simulink library "Simple_lib"  (R2018b)
settings: Solver=ode45  StartTime=0.0  StopTime=10.0  RelTol=1e-3  EnableMultiTasking=on
undefined symbols (not defined in the file or in its folder): Acceptance, beta, C, C_J, C_P, c_wall, dGain, DiscIntNeverNeededParam, Duplex, Electrical_lib, grab, h_fe, i, i3, K_T, Kman, KmanCE, mu_s, n_rev, R_arm, Simplex, systemTs, tau_0, TinIC, Ts, w_0, wallMass, Watch_lib
libraries: $bdroot x407, PlantUtilityBlockset_lib x30, peGeneralControl x22, simulink x11
(part 11 of 14)

== system Simple_lib/Electrical/B2/C ==
  1/C_J : Gain  Gain=1/C_J
  Discrete-Time Integrator1 : DiscreteIntegrator  gainval=1  SampleTime=Ts  ICPrevOutput=DiscIntNeverNeededParam  ICPrevScaledInput=DiscIntNeverNeededParam
  Duplex : Subsystem  AncestorBlock=Electrical_lib/Duplex  InitFcn=bond
      mask Display:
      | plot([1 1], [2 -2])
      | plot([0 1],[0 1])
  J1 : Outport
  wires:
  Discrete-Time Integrator1/1 -> Duplex/1(potential)
  1/C_J/1 -> Discrete-Time Integrator1/1
  Duplex/2(flow) -> 1/C_J/1
  Duplex/1(duplex) -> J1/1

== system Simple_lib/Electrical/B2/E ==
  In1 : Inport
  Constant : Constant  Value=1.5
  Duplex : Subsystem  AncestorBlock=Electrical_lib/Duplex  InitFcn=bond
      mask Display:
      | plot([1 1], [2 -2])
      | plot([0 1],[0 1])
  Simplex : Subsystem  AncestorBlock=Electrical_lib/Simplex  InitFcn=bond
      mask Display:
      | color('white')
      | plot([0 1], [2 2])
      | plot([0 1], [-2 -2])
      | color('black')
      | %patch([0 1 0 0], [0 1 2 0], [0 0 0])
      | plot([0 0], [2 -2])
      | %patch([0 1 1 0 0], [0 0 -2 -2 0], [0 0 0])
      | %patch([-1 0 0 -1 -1], [-2 -2 2 2 -2], [0 0 0])
      | plot([0 1],[1 0])
  Sum : Sum  Inputs=|++
  Out1 : Outport
  wires:
  In1/1 -> Simplex/1(duplex)
  Sum/1 -> Duplex/1(potential)
  Constant/1 -> Sum/2
  Duplex/2(flow) -> Simplex/2(In2)
  Simplex/1(simplex) -> Sum/1
  Duplex/1(duplex) -> Out1/1

== system Simple_lib/Electrical/B2/L ==
  In1 : Inport
  In2 : Inport  Port=2
  1/L : Gain  Gain=-1/1e-1
  1/R2 : Gain  Gain=-1
  1/R3 : Gain  Gain=-1
  Discrete-Time Integrator1 : DiscreteIntegrator  gainval=1  SampleTime=Ts  ICPrevOutput=DiscIntNeverNeededParam  ICPrevScaledInput=DiscIntNeverNeededParam
  Simplex : Subsystem  AncestorBlock=Electrical_lib/Simplex  InitFcn=bond
      mask Display:
      | color('white')
      | plot([0 1], [2 2])
      | plot([0 1], [-2 -2])
      | color('black')
      | %patch([0 1 0 0], [0 1 2 0], [0 0 0])
      | plot([0 0], [2 -2])
      | %patch([0 1 1 0 0], [0 0 -2 -2 0], [0 0 0])
      | %patch([-1 0 0 -1 -1], [-2 -2 2 2 -2], [0 0 0])
      | plot([0 1],[1 0])
  Simplex1 : Subsystem  AncestorBlock=Electrical_lib/Simplex  InitFcn=bond
      mask Display:
      | color('white')
      | plot([0 1], [2 2])
      | plot([0 1], [-2 -2])
      | color('black')
      | %patch([0 1 0 0], [0 1 2 0], [0 0 0])
      | plot([0 0], [2 -2])
      | %patch([0 1 1 0 0], [0 0 -2 -2 0], [0 0 0])
      | %patch([-1 0 0 -1 -1], [-2 -2 2 2 -2], [0 0 0])
      | plot([0 1],[1 0])
  Sum : Sum  Inputs=+|+
  wires:
  In1/1 -> Simplex/1(duplex)
  In2/1 -> Simplex1/1(duplex)
  Sum/1 -> Discrete-Time Integrator1/1
  1/R2/1 -> Sum/1
  1/L/1 -> 1/R3/1, Simplex/2(In2)
  Discrete-Time Integrator1/1 -> 1/L/1
  1/R3/1 -> Simplex1/2(In2)
  Simplex1/1(simplex) -> Sum/2
  Simplex/1(simplex) -> 1/R2/1

== system Simple_lib/Electrical/B2/R0 ==
  In1 : Inport
  Duplex : Subsystem  AncestorBlock=Electrical_lib/Duplex  InitFcn=bond
      mask Display:
      | plot([1 1], [2 -2])
      | plot([0 1],[0 1])
  Gain : Gain  Gain=-1
  Simplex : Subsystem  AncestorBlock=Electrical_lib/Simplex  InitFcn=bond
      mask Display:
      | color('white')
      | plot([0 1], [2 2])
      | plot([0 1], [-2 -2])
      | color('black')
      | %patch([0 1 0 0], [0 1 2 0], [0 0 0])
      | plot([0 0], [2 -2])
      | %patch([0 1 1 0 0], [0 0 -2 -2 0], [0 0 0])
      | %patch([-1 0 0 -1 -1], [-2 -2 2 2 -2], [0 0 0])
      | plot([0 1],[1 0])
  Sum : Sum  Inputs=|++
  resistance : Gain  Gain=R
  Out1 : Outport
  wires:
  Sum/1 -> Duplex/1(potential)
  Gain/1 -> Sum/2
  resistance/1 -> Gain/1
  Duplex/1(duplex) -> Out1/1
  In1/1 -> Simplex/1(duplex)
  Simplex/1(simplex) -> Sum/1
  Duplex/2(flow) -> Simplex/2(In2), resistance/1

== system Simple_lib/Electrical/BiGain/_out ==
  note: {\bf\_out - buses out and logs the signals from the generic {\itOutflow} block}
      |
      | The init function {\itinit\_out} sets up the logging.
  in : Inport  Tag=NOFLUX
  Bus Creator : BusCreator  Inputs=3
  Constant : Constant  Value=[0;0;0]
  Demux : Demux  Outputs=3
  Outflow : $bdroot/Utility/Outflow  Tag=Electrical  SystemSampleTime=-1
  Sum : Sum  Inputs=|++
  Sum2 : Sum  Inputs=+  CollapseMode=Specified dimension  CollapseDim=2
  out : Outport
  backs : Outport  Tag=NOFLUX  Port=2
  wires:
  Demux/3 -> Bus Creator/3  "C"
  Outflow/1 -> out/1
  Bus Creator/1 -> backs/1
  in/1 -> Outflow/1  "V"
  Outflow/2 -> Sum2/1
  Demux/1 -> Bus Creator/1  "I"
  Demux/2 -> Bus Creator/2  "G"
  Sum2/1 -> Sum/1
  Sum/1 -> Demux/1
  Constant/1 -> Sum/2

== system Simple_lib/Electrical/H/Switch Volts ==
  u : Inport
  Sw : Inport  Port=2
  v : Inport  Port=3
  Switch : Switch  Criteria=u2 > Threshold
  Switch1 : Switch
  uSw : Outport
  vSw : Outport  Port=2
  wires:
  u/1 -> Switch/1, Switch1/3
  v/1 -> Switch/3, Switch1/1
  Sw/1 -> Switch/2, Switch1/2
  Switch1/1 -> vSw/1
  Switch/1 -> uSw/1

== system Simple_lib/Electrical/NPN/Transistor Action ==
  Constant : Constant  Value=-0.7
  Gain : Gain  Gain=beta
  Gain1 : Gain  Gain=1/KmanCE
  Gain2 : Gain  Gain=-1/Ts
  Scope : Scope  NumInputPorts=4
  Sum : Sum  Inputs=+|-
  _1 : $bdroot/Utility/Output  Tag=Electrical  Level=Level  Flow=flow
  _2 : $bdroot/Utility/Output  Tag=Electrical  Level=Level  Flow=flow
  dV_BE : Outport
  dV_CE : Outport  Port=2
  wires:
  Constant/1 -> _1/1
  _2/1 -> dV_CE/1
  _1/1 -> dV_BE/1
  Gain2/1 -> Scope/1, _2/1  "dV"
  Gain1/1 -> Gain2/1
  Sum/1 -> Gain1/1, Scope/2  "deltaI"
  _1/2 -> Gain/1
  Gain/1 -> Scope/4, Sum/2  "betaI_BE"
  _2/2 -> Sum/1

== system Simple_lib/Electrical/QTM/TransistorMan ==
  I_B : Inport
  I_C : Inport  Port=2
  DI : Scope
  Discrete-Time Integrator : DiscreteIntegrator  gainval=Kman  SampleTime=-1  LimitOutput=on  LowerSaturationLimit=0  ICPrevOutput=DiscIntNeverNeededParam  ICPrevScaledInput=DiscIntNeverNeededParam
  Gain : Gain  Gain=h_fe
  I_B_ : Scope
  I_C_ : Scope
  Resistance : Scope
  Sum : Sum  Inputs=|+-
  R : Outport
  wires:
  I_C/1 -> I_C_/1, Sum/1
  Gain/1 -> Sum/2
  Discrete-Time Integrator/1 -> Resistance/1, R/1
  Sum/1 -> Discrete-Time Integrator/1, DI/1
  I_B/1 -> I_B_/1, Gain/1

== system Simple_lib/Electrical/R2/Simplex ==
  InPot : Inport
  InFlow : Inport  Tag=NOFLUX  Port=2
  FlowDisplay : Display
  Flow_SimplexR1Inverter_test0 : Scope
      settings: Tag=Flow
  PotDisplay : Display
  Pot_SimplexR1Inverter_test0 : Scope
      settings: Tag=Pot
  Rate Transition : RateTransition  OutPortSampleTimeMultiple=Ts  OutPortSampleTime=Ts
  OutPot : Outport  Tag=NOFLUX
  tag scope: SimplexR1Inverter_test0=global
  wires:
  Rate Transition/1 -> PotDisplay/1, Pot_SimplexR1Inverter_test0/1, OutPot/1
  InFlow/1 -> [SimplexR1Inverter_test0], FlowDisplay/1, Flow_SimplexR1Inverter_test0/1
  InPot/1 -> Rate Transition/1

== system Simple_lib/Electrical/R2/Simplex1 ==
  InPot : Inport
  InFlow : Inport  Tag=NOFLUX  Port=2
  FlowDisplay : Display
  Flow_Simplex1R1Inverter_test0 : Scope
      settings: Tag=Flow
  PotDisplay : Display
  Pot_Simplex1R1Inverter_test0 : Scope
      settings: Tag=Pot
  Rate Transition : RateTransition  OutPortSampleTimeMultiple=Ts  OutPortSampleTime=Ts
  OutPot : Outport  Tag=NOFLUX
  tag scope: Simplex1R1Inverter_test0=global
  wires:
  Rate Transition/1 -> PotDisplay/1, Pot_Simplex1R1Inverter_test0/1, OutPot/1
  InFlow/1 -> [Simplex1R1Inverter_test0], FlowDisplay/1, Flow_Simplex1R1Inverter_test0/1
  InPot/1 -> Rate Transition/1

== system Simple_lib/Electrical/SimplestEMachine/Inertia ==
  note: Differentiate safely
  In1 : Inport
  1/R2 : Gain  Gain=-1
  BigGain : Gain  Gain=dGain
  DB.Dln.ERADEMInertia : Gain  Gain=0.034
  Discrete-Time Integrator1 : DiscreteIntegrator  gainval=1  SampleTime=Ts  ICPrevOutput=DiscIntNeverNeededParam  ICPrevScaledInput=DiscIntNeverNeededParam
  Push : Subsystem  AncestorBlock=PlantUtilityBlockset_lib/Utility/Push  InitFcn=initSimplex
      mask Display:
      | color('white')
      | plot([0 3], [2 2])
      | plot([0 3], [-2 -2])
      | color('black')
      | 
      | plot([0 2 2 3], [1 1 0 0])
      | plot([1 3 2 1 0 2], [0.6 0.6 0.4 0.6 0.4 0.4])
      | patch([1 3 2],[0.6 0.6 0.4],[0,0,0])
      | plot([0 1 1], [1 1 0.6])
      | plot([1 1 0], [0.4 -1 -1])
  Sum : Sum  Inputs=|++
  wires:
  Sum/1 -> BigGain/1
  Discrete-Time Integrator1/1 -> 1/R2/1
  BigGain/1 -> DB.Dln.ERADEMInertia/1, Discrete-Time Integrator1/1
  DB.Dln.ERADEMInertia/1 -> Push/2(InFlow)
  1/R2/1 -> Sum/2
  Push/1(OutPot) -> Sum/1
  In1/1 -> Push/1(InPot)

== system Simple_lib/Electrical/SimplestEMachine/Transducer ==
  w : Inport
  Duplex : Subsystem  Tag=Electrical  AncestorBlock=PlantUtilityBlockset_lib/Utility/Pull  InitFcn=initDuplex
      mask Display:
      | color('white')
      | plot([0 3], [2 2])
      | plot([0 3], [-2 -2])
      | color('black')
      | 
      | plot([0 1 1], [0 0 0.4])
      | plot([1 1 3], [0.6 1 1])
      | plot([1 3 2 1 0 2], [0.6 0.6 0.4 0.6 0.4 0.4])
      | patch([0 2 1],[0.4 0.4 0.6],[0,0,0])
      | plot([3 2 2], [1 1 0.6])
      | plot([2 2 3], [0.4 -1 -1])
  Simplex : Subsystem  Tag=Electrical  AncestorBlock=PlantUtilityBlockset_lib/Utility/Push  InitFcn=initSimplex
      mask Display:
      | color('white')
      | plot([0 3], [2 2])
      | plot([0 3], [-2 -2])
      | color('black')
      | 
      | plot([0 2 2 3], [1 1 0 0])
      | plot([1 3 2 1 0 2], [0.6 0.6 0.4 0.6 0.4 0.4])
      | patch([1 3 2],[0.6 0.6 0.4],[0,0,0])
      | plot([0 1 1], [1 1 0.6])
      | plot([1 1 0], [0.4 -1 -1])
  Torque Constant = 60/2/pi/K_V : Gain  Gain=K_T
  Torque Constant K_T : Gain  Gain=K_T
  V : Outport
  wires:
  Torque Constant K_T/1 -> Simplex/2(InFlow)  "tau"
  Simplex/1(OutPot) -> Torque Constant = 60/2/pi/K_V/1
  Duplex/1(OutPot) -> V/1
  w/1 -> Simplex/1(InPot)
  Duplex/2(OutFlow) -> Torque Constant K_T/1  "I"
  Torque Constant = 60/2/pi/K_V/1 -> Duplex/1(InPot)

== system Simple_lib/Electrical/TM/Reverse ==
  Vup : Inport
  Constant : Constant  Value=0.6
  I_out : Scope
  Input : $bdroot/Utility/Input  Level=V  Flow=I
  Sum : Sum  Inputs=|++
  Sum1 : Sum  Inputs=+
  _ : $bdroot/Utility/Output  Tag=Electrical  Level=Level  Flow=flow
  Vdn : Outport
  wires:
  Vup/1 -> Input/1
  Input/1 -> Sum/1
  Sum1/1 -> I_out/1, Input/2
  Sum/1 -> _/1
  _/1 -> Vdn/1
  _/2 -> Sum1/1
  Constant/1 -> Sum/2

== system Simple_lib/Electrical/TM/Rman ==
  In1 : Inport
  In3 : Inport  Port=2
  In2 : Inport  Port=3
  1/R2 : Gain  Gain=-1
  1/R3 : Gain  Gain=-1
  Constant : Constant  Value=i
  Divide : Product  Inputs=**
  Input2 : $bdroot/Utility/Input  Level=V  Flow=I
  Input3 : $bdroot/Utility/Input  Level=V  Flow=I
  Sum : Sum  Inputs=+++
  wires:
  In3/1 -> Divide/2
  Constant/1 -> Sum/2
  1/R3/1 -> Input3/2
  1/R2/1 -> Sum/3
  Divide/1 -> Input2/2, 1/R3/1
  Input2/1 -> Sum/1
  Input3/1 -> 1/R2/1
  In1/1 -> Input2/1
  Sum/1 -> Divide/1
  In2/1 -> Input3/1

== system Simple_lib/Electrical/TM/TransistorMan ==
  I_C : Inport
  I_B : Inport  Port=2
  DI : Scope
  Discrete-Time Integrator : DiscreteIntegrator  gainval=Kman  SampleTime=-1  LimitOutput=on  LowerSaturationLimit=0  ICPrevOutput=DiscIntNeverNeededParam  ICPrevScaledInput=DiscIntNeverNeededParam
  Gain : Gain  Gain=h_fe
  I_B_ : Scope
  I_C_ : Scope
  Sum : Sum  Inputs=|--
  conductance : Scope
  cond : Outport
  wires:
  I_C/1 -> I_C_/1, Sum/1
  Gain/1 -> Sum/2
  Discrete-Time Integrator/1 -> conductance/1, cond/1
  Sum/1 -> Discrete-Time Integrator/1, DI/1
  I_B/1 -> I_B_/1, Gain/1

== system Simple_lib/Electrical/Windings/IM ==
  In1 : Inport
  Duplex : Subsystem  Tag=Electrical  AncestorBlock=PlantUtilityBlockset_lib/Utility/Pull  InitFcn=initDuplex
      mask Display:
      | color('white')
      | plot([0 3], [2 2])
      | plot([0 3], [-2 -2])
      | color('black')
      | 
      | plot([0 1 1], [0 0 0.4])
      | plot([1 1 3], [0.6 1 1])
      | plot([1 3 2 1 0 2], [0.6 0.6 0.4 0.6 0.4 0.4])
      | patch([0 2 1],[0.4 0.4 0.6],[0,0,0])
      | plot([3 2 2], [1 1 0.6])
      | plot([2 2 3], [0.4 -1 -1])
  Simplex : Subsystem  Tag=Electrical  AncestorBlock=PlantUtilityBlockset_lib/Utility/Push  InitFcn=initSimplex
      mask Display:
      | color('white')
      | plot([0 3], [2 2])
      | plot([0 3], [-2 -2])
      | color('black')
      | 
      | plot([0 2 2 3], [1 1 0 0])
      | plot([1 3 2 1 0 2], [0.6 0.6 0.4 0.6 0.4 0.4])
      | patch([1 3 2],[0.6 0.6 0.4],[0,0,0])
      | plot([0 1 1], [1 1 0.6])
      | plot([1 1 0], [0.4 -1 -1])
  Out1 : Outport
  Out2 : Outport  Port=2
  wires:
  In1/1 -> Simplex/1(InPot)
  Duplex/1(OutPot) -> Out1/1
  Duplex/2(OutFlow) -> Simplex/2(InFlow), Out2/1
  Simplex/1(OutPot) -> Duplex/1(InPot)

== system Simple_lib/Electrical/Windings/IM1 ==
  In1 : Inport
  Duplex : Subsystem  Tag=Electrical  AncestorBlock=PlantUtilityBlockset_lib/Utility/Pull  InitFcn=initDuplex
      mask Display:
      | color('white')
      | plot([0 3], [2 2])
      | plot([0 3], [-2 -2])
      | color('black')
      | 
      | plot([0 1 1], [0 0 0.4])
      | plot([1 1 3], [0.6 1 1])
      | plot([1 3 2 1 0 2], [0.6 0.6 0.4 0.6 0.4 0.4])
      | patch([0 2 1],[0.4 0.4 0.6],[0,0,0])
      | plot([3 2 2], [1 1 0.6])
      | plot([2 2 3], [0.4 -1 -1])
  Simplex : Subsystem  Tag=Electrical  AncestorBlock=PlantUtilityBlockset_lib/Utility/Push  InitFcn=initSimplex
      mask Display:
      | color('white')
      | plot([0 3], [2 2])
      | plot([0 3], [-2 -2])
      | color('black')
      | 
      | plot([0 2 2 3], [1 1 0 0])
      | plot([1 3 2 1 0 2], [0.6 0.6 0.4 0.6 0.4 0.4])
      | patch([1 3 2],[0.6 0.6 0.4],[0,0,0])
      | plot([0 1 1], [1 1 0.6])
      | plot([1 1 0], [0.4 -1 -1])
  Out1 : Outport
  Out2 : Outport  Port=2
  wires:
  In1/1 -> Simplex/1(InPot)
  Duplex/1(OutPot) -> Out1/1
  Duplex/2(OutFlow) -> Simplex/2(InFlow), Out2/1
  Simplex/1(OutPot) -> Duplex/1(InPot)

== system Simple_lib/Electrical/Windings/IM2 ==
  In1 : Inport
  Duplex : Subsystem  Tag=Electrical  AncestorBlock=PlantUtilityBlockset_lib/Utility/Pull  InitFcn=initDuplex
      mask Display:
      | color('white')
      | plot([0 3], [2 2])
      | plot([0 3], [-2 -2])
      | color('black')
      | 
      | plot([0 1 1], [0 0 0.4])
      | plot([1 1 3], [0.6 1 1])
      | plot([1 3 2 1 0 2], [0.6 0.6 0.4 0.6 0.4 0.4])
      | patch([0 2 1],[0.4 0.4 0.6],[0,0,0])
      | plot([3 2 2], [1 1 0.6])
      | plot([2 2 3], [0.4 -1 -1])
  Simplex : Subsystem  Tag=Electrical  AncestorBlock=PlantUtilityBlockset_lib/Utility/Push  InitFcn=initSimplex
      mask Display:
      | color('white')
      | plot([0 3], [2 2])
      | plot([0 3], [-2 -2])
      | color('black')
      | 
      | plot([0 2 2 3], [1 1 0 0])
      | plot([1 3 2 1 0 2], [0.6 0.6 0.4 0.6 0.4 0.4])
      | patch([1 3 2],[0.6 0.6 0.4],[0,0,0])
      | plot([0 1 1], [1 1 0.6])
      | plot([1 1 0], [0.4 -1 -1])
  Out1 : Outport
  Out2 : Outport  Port=2
  wires:
  In1/1 -> Simplex/1(InPot)
  Duplex/1(OutPot) -> Out1/1
  Duplex/2(OutFlow) -> Simplex/2(InFlow), Out2/1
  Simplex/1(OutPot) -> Duplex/1(InPot)

== system Simple_lib/Electrical/Windings/L1 ==
  In1 : Inport
  In2 : Inport  Port=2
  1/R1 : Gain  Gain=-1
  1/R2 : Gain  Gain=-1
  1/R3 : Gain  Gain=-1/L
  Discrete-Time Integrator1 : DiscreteIntegrator  gainval=1  SampleTime=Ts  ICPrevOutput=DiscIntNeverNeededParam  ICPrevScaledInput=DiscIntNeverNeededParam
  Simplex : Subsystem  AncestorBlock=PlantUtilityBlockset_lib/Utility/Push  InitFcn=initSimplex
      mask Display:
      | color('white')
      | plot([0 3], [2 2])
      | plot([0 3], [-2 -2])
      | color('black')
      | 
      | plot([0 2 2 3], [1 1 0 0])
      | plot([1 3 2 1 0 2], [0.6 0.6 0.4 0.6 0.4 0.4])
      | patch([1 3 2],[0.6 0.6 0.4],[0,0,0])
      | plot([0 1 1], [1 1 0.6])
      | plot([1 1 0], [0.4 -1 -1])
  Simplex1 : Subsystem  AncestorBlock=PlantUtilityBlockset_lib/Utility/Push  InitFcn=initSimplex
      mask Display:
      | color('white')
      | plot([0 3], [2 2])
      | plot([0 3], [-2 -2])
      | color('black')
      | 
      | plot([0 2 2 3], [1 1 0 0])
      | plot([1 3 2 1 0 2], [0.6 0.6 0.4 0.6 0.4 0.4])
      | patch([1 3 2],[0.6 0.6 0.4],[0,0,0])
      | plot([0 1 1], [1 1 0.6])
      | plot([1 1 0], [0.4 -1 -1])
  Sum : Sum  Inputs=+|+
  wires:
  1/R1/1 -> Simplex1/2(InFlow)
  Simplex1/1(OutPot) -> Sum/2
  In2/1 -> Simplex1/1(InPot)
  Sum/1 -> Discrete-Time Integrator1/1
  1/R2/1 -> Sum/1
  Simplex/1(OutPot) -> 1/R2/1
  In1/1 -> Simplex/1(InPot)
  Discrete-Time Integrator1/1 -> 1/R3/1
  1/R3/1 -> 1/R1/1, Simplex/2(InFlow)

== system Simple_lib/Electrical/Windings/L2 ==
  In1 : Inport
  In2 : Inport  Port=2
  1/R1 : Gain  Gain=-1
  1/R2 : Gain  Gain=-1
  1/R3 : Gain  Gain=-1/L
  Discrete-Time Integrator1 : DiscreteIntegrator  gainval=1  SampleTime=Ts  ICPrevOutput=DiscIntNeverNeededParam  ICPrevScaledInput=DiscIntNeverNeededParam
  Simplex : Subsystem  AncestorBlock=PlantUtilityBlockset_lib/Utility/Push  InitFcn=initSimplex
      mask Display:
      | color('white')
      | plot([0 3], [2 2])
      | plot([0 3], [-2 -2])
      | color('black')
      | 
      | plot([0 2 2 3], [1 1 0 0])
      | plot([1 3 2 1 0 2], [0.6 0.6 0.4 0.6 0.4 0.4])
      | patch([1 3 2],[0.6 0.6 0.4],[0,0,0])
      | plot([0 1 1], [1 1 0.6])
      | plot([1 1 0], [0.4 -1 -1])
  Simplex1 : Subsystem  AncestorBlock=PlantUtilityBlockset_lib/Utility/Push  InitFcn=initSimplex
      mask Display:
      | color('white')
      | plot([0 3], [2 2])
      | plot([0 3], [-2 -2])
      | color('black')
      | 
      | plot([0 2 2 3], [1 1 0 0])
      | plot([1 3 2 1 0 2], [0.6 0.6 0.4 0.6 0.4 0.4])
      | patch([1 3 2],[0.6 0.6 0.4],[0,0,0])
      | plot([0 1 1], [1 1 0.6])
      | plot([1 1 0], [0.4 -1 -1])
  Sum : Sum  Inputs=+|+
  wires:
  1/R1/1 -> Simplex1/2(InFlow)
  Simplex1/1(OutPot) -> Sum/2
  In2/1 -> Simplex1/1(InPot)
  Sum/1 -> Discrete-Time Integrator1/1
  1/R2/1 -> Sum/1
  Simplex/1(OutPot) -> 1/R2/1
  In1/1 -> Simplex/1(InPot)
  Discrete-Time Integrator1/1 -> 1/R3/1
  1/R3/1 -> 1/R1/1, Simplex/2(InFlow)

== system Simple_lib/Electrical/Windings/L3 ==
  In1 : Inport
  In2 : Inport  Port=2
  1/R1 : Gain  Gain=-1
  1/R2 : Gain  Gain=-1
  1/R3 : Gain  Gain=-1/L
  Discrete-Time Integrator1 : DiscreteIntegrator  gainval=1  SampleTime=Ts  ICPrevOutput=DiscIntNeverNeededParam  ICPrevScaledInput=DiscIntNeverNeededParam
  Simplex : Subsystem  AncestorBlock=PlantUtilityBlockset_lib/Utility/Push  InitFcn=initSimplex
      mask Display:
      | color('white')
      | plot([0 3], [2 2])
      | plot([0 3], [-2 -2])
      | color('black')
      | 
      | plot([0 2 2 3], [1 1 0 0])
      | plot([1 3 2 1 0 2], [0.6 0.6 0.4 0.6 0.4 0.4])
      | patch([1 3 2],[0.6 0.6 0.4],[0,0,0])
      | plot([0 1 1], [1 1 0.6])
      | plot([1 1 0], [0.4 -1 -1])
  Simplex1 : Subsystem  AncestorBlock=PlantUtilityBlockset_lib/Utility/Push  InitFcn=initSimplex
      mask Display:
      | color('white')
      | plot([0 3], [2 2])
      | plot([0 3], [-2 -2])
      | color('black')
      | 
      | plot([0 2 2 3], [1 1 0 0])
      | plot([1 3 2 1 0 2], [0.6 0.6 0.4 0.6 0.4 0.4])
      | patch([1 3 2],[0.6 0.6 0.4],[0,0,0])
      | plot([0 1 1], [1 1 0.6])
      | plot([1 1 0], [0.4 -1 -1])
  Sum : Sum  Inputs=+|+
  wires:
  1/R1/1 -> Simplex1/2(InFlow)
  Simplex1/1(OutPot) -> Sum/2
  In2/1 -> Simplex1/1(InPot)
  Sum/1 -> Discrete-Time Integrator1/1
  1/R2/1 -> Sum/1
  Simplex/1(OutPot) -> 1/R2/1
  In1/1 -> Simplex/1(InPot)
  Discrete-Time Integrator1/1 -> 1/R3/1
  1/R3/1 -> 1/R1/1, Simplex/2(InFlow)

== system Simple_lib/Electrical/Windings/R ==
  In1 : Inport
  Duplex : Subsystem  Tag=Electrical  AncestorBlock=PlantUtilityBlockset_lib/Utility/Pull  InitFcn=initDuplex
      mask Display:
      | color('white')
      | plot([0 3], [2 2])
      | plot([0 3], [-2 -2])
      | color('black')
      | 
      | plot([0 1 1], [0 0 0.4])
      | plot([1 1 3], [0.6 1 1])
      | plot([1 3 2 1 0 2], [0.6 0.6 0.4 0.6 0.4 0.4])
      | patch([0 2 1],[0.4 0.4 0.6],[0,0,0])
      | plot([3 2 2], [1 1 0.6])
      | plot([2 2 3], [0.4 -1 -1])
  Simplex : Subsystem  Tag=Electrical  AncestorBlock=PlantUtilityBlockset_lib/Utility/Push  InitFcn=initSimplex
      mask Display:
      | color('white')
      | plot([0 3], [2 2])
      | plot([0 3], [-2 -2])
      | color('black')
      | 
      | plot([0 2 2 3], [1 1 0 0])
      | plot([1 3 2 1 0 2], [0.6 0.6 0.4 0.6 0.4 0.4])
      | patch([1 3 2],[0.6 0.6 0.4],[0,0,0])
      | plot([0 1 1], [1 1 0.6])
      | plot([1 1 0], [0.4 -1 -1])
  Sum : Sum  Inputs=|++
  resistance : Gain  Gain=R
  Out1 : Outport
  wires:
  In1/1 -> Simplex/1(InPot)
  Duplex/1(OutPot) -> Out1/1
  Duplex/2(OutFlow) -> Simplex/2(InFlow), resistance/1
  Simplex/1(OutPot) -> Sum/1
  resistance/1 -> Sum/2
  Sum/1 -> Duplex/1(InPot)

== system Simple_lib/Electrical/Windings/R1 ==
  In1 : Inport
  Duplex : Subsystem  Tag=Electrical  AncestorBlock=PlantUtilityBlockset_lib/Utility/Pull  InitFcn=initDuplex
      mask Display:
      | color('white')
      | plot([0 3], [2 2])
      | plot([0 3], [-2 -2])
      | color('black')
      | 
      | plot([0 1 1], [0 0 0.4])
      | plot([1 1 3], [0.6 1 1])
      | plot([1 3 2 1 0 2], [0.6 0.6 0.4 0.6 0.4 0.4])
      | patch([0 2 1],[0.4 0.4 0.6],[0,0,0])
      | plot([3 2 2], [1 1 0.6])
      | plot([2 2 3], [0.4 -1 -1])
  Simplex : Subsystem  Tag=Electrical  AncestorBlock=PlantUtilityBlockset_lib/Utility/Push  InitFcn=initSimplex
      mask Display:
      | color('white')
      | plot([0 3], [2 2])
      | plot([0 3], [-2 -2])
      | color('black')
      | 
      | plot([0 2 2 3], [1 1 0 0])
      | plot([1 3 2 1 0 2], [0.6 0.6 0.4 0.6 0.4 0.4])
      | patch([1 3 2],[0.6 0.6 0.4],[0,0,0])
      | plot([0 1 1], [1 1 0.6])
      | plot([1 1 0], [0.4 -1 -1])
  Sum : Sum  Inputs=|++
  resistance : Gain  Gain=R
  Out1 : Outport
  wires:
  In1/1 -> Simplex/1(InPot)
  Duplex/1(OutPot) -> Out1/1
  Duplex/2(OutFlow) -> Simplex/2(InFlow), resistance/1
  Simplex/1(OutPot) -> Sum/1
  resistance/1 -> Sum/2
  Sum/1 -> Duplex/1(InPot)

== system Simple_lib/Electrical/Windings/R2 ==
  In1 : Inport
  Duplex : Subsystem  Tag=Electrical  AncestorBlock=PlantUtilityBlockset_lib/Utility/Pull  InitFcn=initDuplex
      mask Display:
      | color('white')
      | plot([0 3], [2 2])
      | plot([0 3], [-2 -2])
      | color('black')
      | 
      | plot([0 1 1], [0 0 0.4])
      | plot([1 1 3], [0.6 1 1])
      | plot([1 3 2 1 0 2], [0.6 0.6 0.4 0.6 0.4 0.4])
      | patch([0 2 1],[0.4 0.4 0.6],[0,0,0])
      | plot([3 2 2], [1 1 0.6])
      | plot([2 2 3], [0.4 -1 -1])
  Simplex : Subsystem  Tag=Electrical  AncestorBlock=PlantUtilityBlockset_lib/Utility/Push  InitFcn=initSimplex
      mask Display:
      | color('white')
      | plot([0 3], [2 2])
      | plot([0 3], [-2 -2])
      | color('black')
      | 
      | plot([0 2 2 3], [1 1 0 0])
      | plot([1 3 2 1 0 2], [0.6 0.6 0.4 0.6 0.4 0.4])
      | patch([1 3 2],[0.6 0.6 0.4],[0,0,0])
      | plot([0 1 1], [1 1 0.6])
      | plot([1 1 0], [0.4 -1 -1])
  Sum : Sum  Inputs=|++
  resistance : Gain  Gain=R
  Out1 : Outport
  wires:
  In1/1 -> Simplex/1(InPot)
  Duplex/1(OutPot) -> Out1/1
  Duplex/2(OutFlow) -> Simplex/2(InFlow), resistance/1
  Simplex/1(OutPot) -> Sum/1
  resistance/1 -> Sum/2
  Sum/1 -> Duplex/1(InPot)

== system Simple_lib/Electrical/Windings/Va ==
  InPot : Inport  Tag=NOFLUX
  FlowDisplay : Display
  FlowGain : Gain
  Flow_VaWindingsMk4v3Inverter_test0 : Scope
      settings: Tag=Flow
  PotDisplay : Display
  Pot_VaWindingsMk4v3Inverter_test0 : Scope
      settings: Tag=Pot
  Rate Transition : RateTransition  OutPortSampleTimeMultiple=nT  OutPortSampleTime=Ts
  OutPot : Outport
  OutFlow : Outport  Tag=NOFLUX  Port=2
  wires:
  Rate Transition/1 -> OutPot/1
  InPot/1 -> Rate Transition/1, PotDisplay/1, Pot_VaWindingsMk4v3Inverter_test0/1
  FlowGain/1 -> OutFlow/1, FlowDisplay/1, Flow_VaWindingsMk4v3Inverter_test0/1
  [SimplexRWindingsMk4v3Inverter_test0] -> FlowGain/1

== system Simple_lib/Electrical/Windings/Vb ==
  InPot : Inport  Tag=NOFLUX
  FlowDisplay : Display
  FlowGain : Gain
  Flow_VbWindingsMk4v3Inverter_test0 : Scope
      settings: Tag=Flow
  PotDisplay : Display
  Pot_VbWindingsMk4v3Inverter_test0 : Scope
      settings: Tag=Pot
  Rate Transition : RateTransition  OutPortSampleTimeMultiple=nT  OutPortSampleTime=Ts
  OutPot : Outport
  OutFlow : Outport  Tag=NOFLUX  Port=2
  wires:
  Rate Transition/1 -> OutPot/1
  InPot/1 -> Rate Transition/1, PotDisplay/1, Pot_VbWindingsMk4v3Inverter_test0/1
  FlowGain/1 -> OutFlow/1, FlowDisplay/1, Flow_VbWindingsMk4v3Inverter_test0/1
  [SimplexR1WindingsMk4v3Inverter_test0] -> FlowGain/1

== system Simple_lib/Electrical/Windings/Vc ==
  InPot : Inport  Tag=NOFLUX
  FlowDisplay : Display
  FlowGain : Gain
  Flow_VcWindingsMk4v3Inverter_test0 : Scope
      settings: Tag=Flow
  PotDisplay : Display
  Pot_VcWindingsMk4v3Inverter_test0 : Scope
      settings: Tag=Pot
  Rate Transition : RateTransition  OutPortSampleTimeMultiple=nT  OutPortSampleTime=Ts
  OutPot : Outport
  OutFlow : Outport  Tag=NOFLUX  Port=2
  wires:
  Rate Transition/1 -> OutPot/1
  InPot/1 -> Rate Transition/1, PotDisplay/1, Pot_VcWindingsMk4v3Inverter_test0/1
  FlowGain/1 -> OutFlow/1, FlowDisplay/1, Flow_VcWindingsMk4v3Inverter_test0/1
  [SimplexR2WindingsMk4v3Inverter_test0] -> FlowGain/1

== system Simple_lib/Electronics/BiGain/_out ==
  note: {\bf\_out - buses out and logs the signals from the generic {\itOutflow} block}
      |
      | The init function {\itinit\_out} sets up the logging.
  in : Inport  Tag=NOFLUX
  Bus Creator : BusCreator  Inputs=3
  Constant : Constant  Value=[0;0;0]
  Demux : Demux  Outputs=3
  Outflow : $bdroot/Utility/Outflow  Tag=Electrical  SystemSampleTime=-1
  Sum : Sum  Inputs=|++
  Sum2 : Sum  Inputs=+  CollapseMode=Specified dimension  CollapseDim=2
  out : Outport
  backs : Outport  Tag=NOFLUX  Port=2
  wires:
  Demux/3 -> Bus Creator/3  "C"
  Outflow/1 -> out/1
  Bus Creator/1 -> backs/1
  in/1 -> Outflow/1  "V"
  Outflow/2 -> Sum2/1
  Demux/1 -> Bus Creator/1  "I"
  Demux/2 -> Bus Creator/2  "G"
  Sum2/1 -> Sum/1
  Sum/1 -> Demux/1
  Constant/1 -> Sum/2

== system Simple_lib/Electronics/NPN_SimpleRR/TransistorMan ==
  Collector : Inport
  I : Inport  Port=2
  Emitter : Inport  Port=3
  Bus Creator : BusCreator  Inputs=3
  Bus Creator1 : BusCreator  Inputs=3
  Constant : Constant  Value=99
  Constant1 : Constant  Value=99
  Cosh : Trigonometry  Operator=cosh
  Gain : Gain  Gain=-1
  Gain1 : Gain  Gain=-1
  Gain2 : Gain
  Gain3 : Gain
  Ground1 : Ground
  Multiply : Product  Inputs=3
  Multiply1 : Product  Inputs=*//*
  Saturation : Saturate  UpperLimit=inf  LowerLimit=-inf
  Sum : Sum  Inputs=+|-
  Tanh : Trigonometry  Operator=tanh
  _Col : $bdroot/Electronics/_in  Level=V  Flow=I
  _Em : $bdroot/Electronics/_in  Level=V  Flow=I
  wires:
  I/1 -> Gain1/1
  Gain3/1 -> Bus Creator/1  "I"
  Gain2/1 -> Bus Creator1/2  "G"
  Gain1/1 -> Saturation/1  "I"
  Saturation/1 -> Multiply/1, Multiply1/4
  Constant1/1 -> Multiply1/1
  Multiply1/1 -> Bus Creator/2, Gain2/1  "G"
  Cosh/1 -> Multiply1/3, Multiply1/2
  Bus Creator/1 -> _Col/2
  Bus Creator1/1 -> _Em/2
  Ground1/1 -> Bus Creator/3, Bus Creator1/1  "C"
  Gain/1 -> Bus Creator1/3  "I"
  Multiply/1 -> Gain/1, Gain3/1  "I"
  Constant/1 -> Multiply/3
  Tanh/1 -> Multiply/2
  Sum/1 -> Tanh/1, Cosh/1
  _Em/1 -> Sum/2
  Emitter/1 -> _Em/1
  _Col/1 -> Sum/1
  Collector/1 -> _Col/1

== system Simple_lib/Electronics/Rnl1/Derivative ==
  y : Inport
  x : Inport  Port=2
  Abs : Abs
  Divide : Product  Inputs=*/
  Ground{1..4} (4 alike) : Ground
  Integrator (Discrete or Continuous)1 : peGeneralControl/Integrator (Discrete or Continuous)  LabelModeActiveChoice=Discrete  ExternalReset=level  LimitType=Anti-windup  B=inf  A=-inf  Ts=-1
  Integrator (Discrete or Continuous)2 : peGeneralControl/Integrator (Discrete or Continuous)  LabelModeActiveChoice=Discrete  ExternalReset=level  LimitType=Anti-windup  B=inf  A=-inf  Ts=-1
  Saturation : Saturate  UpperLimit=inf  LowerLimit=-inf
  Sum1 : Sum  Inputs=|+-
  Sum2 : Sum  Inputs=|+-
  Switch : Switch  Criteria=u2 > Threshold  Threshold=1e-6
  Unit Delay : UnitDelay  SampleTime=-1
  Weighted Sample Time1 : SampleTimeMath  TsampMathOp=/  weightValue=1
  Weighted Sample Time3 : SampleTimeMath  TsampMathOp=/  weightValue=1
  dy/dx : Outport
  wires:
  x/1 -> Sum2/1
  Integrator (Discrete or Continuous)2/1 -> Sum2/2
  Ground1/1 -> Integrator (Discrete or Continuous)2/2
  Sum2/1 -> Weighted Sample Time1/1
  Ground4/1 -> Integrator (Discrete or Continuous)2/3
  Weighted Sample Time1/1 -> Integrator (Discrete or Continuous)2/1, Abs/1, Divide/2  "dI"
  y/1 -> Sum1/1
  Integrator (Discrete or Continuous)1/1 -> Sum1/2
  Ground2/1 -> Integrator (Discrete or Continuous)1/2
  Sum1/1 -> Weighted Sample Time3/1
  Ground3/1 -> Integrator (Discrete or Continuous)1/3
  Weighted Sample Time3/1 -> Integrator (Discrete or Continuous)1/1, Divide/1  "dI"
  Abs/1 -> Switch/2
  Saturation/1 -> dy/dx/1, Unit Delay/1
  Unit Delay/1 -> Switch/3
  Switch/1 -> Saturation/1
  Divide/1 -> Switch/1

== system Simple_lib/Hydraulic/ Heat Exchanger/Linear Heat Pipe ==
  pT_in : Inport
  Gain : Gain  Gain=-1
  Gain1 : Gain  Gain=1e3
  Pull : Subsystem  Tag=Electrical  AncestorBlock=PlantUtilityBlockset_lib/Utility/Pull  InitFcn=initDuplex
      mask Display:
      | color('white')
      | plot([0 3], [2 2])
      | plot([0 3], [-2 -2])
      | color('black')
      | 
      | plot([0 1 1], [0 0 0.4])
      | plot([1 1 3], [0.6 1 1])
      | plot([1 3 2 1 0 2], [0.6 0.6 0.4 0.6 0.4 0.4])
      | patch([0 2 1],[0.4 0.4 0.6],[0,0,0])
      | plot([3 2 2], [1 1 0.6])
      | plot([2 2 3], [0.4 -1 -1])
  Push : Subsystem  AncestorBlock=PlantUtilityBlockset_lib/Utility/Push  InitFcn=initSimplex
      mask Display:
      | color('white')
      | plot([0 3], [2 2])
      | plot([0 3], [-2 -2])
      | color('black')
      | 
      | plot([0 2 2 3], [1 1 0 0])
      | plot([1 3 2 1 0 2], [0.6 0.6 0.4 0.6 0.4 0.4])
      | patch([1 3 2],[0.6 0.6 0.4],[0,0,0])
      | plot([0 1 1], [1 1 0.6])
      | plot([1 1 0], [0.4 -1 -1])
  Sum : Sum  Inputs=|++
  pT_out : Outport
  wires:
  pT_in/1 -> Push/1(InPot)
  Pull/1(OutPot) -> pT_out/1
  Gain1/1 -> Gain/1
  Pull/2(OutFlow) -> Gain1/1, Push/2(InFlow)
  Gain/1 -> Sum/2
  Sum/1 -> Pull/1(InPot)
  Push/1(OutPot) -> Sum/1

== system Simple_lib/Hydraulic/ Heat Exchanger/Linear Heat Pipe1 ==
  pT_in : Inport
  Gain : Gain  Gain=-1
  Gain1 : Gain  Gain=1e3
  Pull : Subsystem  Tag=Electrical  AncestorBlock=PlantUtilityBlockset_lib/Utility/Pull  InitFcn=initDuplex
      mask Display:
      | color('white')
      | plot([0 3], [2 2])
      | plot([0 3], [-2 -2])
      | color('black')
      | 
      | plot([0 1 1], [0 0 0.4])
      | plot([1 1 3], [0.6 1 1])
      | plot([1 3 2 1 0 2], [0.6 0.6 0.4 0.6 0.4 0.4])
      | patch([0 2 1],[0.4 0.4 0.6],[0,0,0])
      | plot([3 2 2], [1 1 0.6])
      | plot([2 2 3], [0.4 -1 -1])
  Push : Subsystem  AncestorBlock=PlantUtilityBlockset_lib/Utility/Push  InitFcn=initSimplex
      mask Display:
      | color('white')
      | plot([0 3], [2 2])
      | plot([0 3], [-2 -2])
      | color('black')
      | 
      | plot([0 2 2 3], [1 1 0 0])
      | plot([1 3 2 1 0 2], [0.6 0.6 0.4 0.6 0.4 0.4])
      | patch([1 3 2],[0.6 0.6 0.4],[0,0,0])
      | plot([0 1 1], [1 1 0.6])
      | plot([1 1 0], [0.4 -1 -1])
  Sum : Sum  Inputs=|++
  pT_out : Outport
  wires:
  pT_in/1 -> Push/1(InPot)
  Pull/1(OutPot) -> pT_out/1
  Gain1/1 -> Gain/1
  Pull/2(OutFlow) -> Gain1/1, Push/2(InFlow)
  Gain/1 -> Sum/2
  Sum/1 -> Pull/1(InPot)
  Push/1(OutPot) -> Sum/1

== system Simple_lib/Hydraulic/Accumulator/Duplex ==
  InPot : Inport  Tag=NOFLUX
  FlowDisplay : Display
  FlowGain : Gain
  Flow_DuplexDivelineDoubleClutch1 : Scope
      settings: Tag=Flow
  PotDisplay : Display
  Pot_DuplexDivelineDoubleClutch1 : Scope
      settings: Tag=Pot
  Rate Transition : RateTransition  OutPortSampleTimeOpt=Multiple of input port sample time  OutPortSampleTimeMultiple=nT
  OutPot : Outport
  OutFlow : Outport  Tag=NOFLUX  Port=2
  wires:
  Rate Transition/1 -> OutPot/1
  InPot/1 -> Rate Transition/1, PotDisplay/1, Pot_DuplexDivelineDoubleClutch1/1
  FlowGain/1 -> OutFlow/1, Flow_DuplexDivelineDoubleClutch1/1, FlowDisplay/1

== system Simple_lib/Hydraulic/Heat Sink/Linear Heat Pipe1 ==
  note: \Delta T = Q / (qc\rho))
  note: \Delta p = - k q
  pT_in : Inport
  Bus Creator1 : BusCreator  Inputs=2
  Bus Selector : BusSelector  OutputSignals=T,p
  Gain : Gain  Gain=-1
  Gain1 : Gain  Gain=1e3
  Product : Product  Inputs=*///
  Pull : Subsystem  Tag=Electrical  AncestorBlock=PlantUtilityBlockset_lib/Utility/Pull  InitFcn=initDuplex
      mask Display:
      | color('white')
      | plot([0 3], [2 2])
      | plot([0 3], [-2 -2])
      | color('black')
      | 
      | plot([0 1 1], [0 0 0.4])
      | plot([1 1 3], [0.6 1 1])
      | plot([1 3 2 1 0 2], [0.6 0.6 0.4 0.6 0.4 0.4])
      | patch([0 2 1],[0.4 0.4 0.6],[0,0,0])
      | plot([3 2 2], [1 1 0.6])
      | plot([2 2 3], [0.4 -1 -1])
  Pull1 : PlantUtilityBlockset_lib/Hydraulic/Linear Heat Pipe/Pull  Tag=Electrical  SystemSampleTime=-1
  Push : Subsystem  AncestorBlock=PlantUtilityBlockset_lib/Utility/Push  InitFcn=initSimplex
      mask Display:
      | color('white')
      | plot([0 3], [2 2])
      | plot([0 3], [-2 -2])
      | color('black')
      | 
      | plot([0 2 2 3], [1 1 0 0])
      | plot([1 3 2 1 0 2], [0.6 0.6 0.4 0.6 0.4 0.4])
      | patch([1 3 2],[0.6 0.6 0.4],[0,0,0])
      | plot([0 1 1], [1 1 0.6])
      | plot([1 1 0], [0.4 -1 -1])
  Sum : Sum  Inputs=|++
  Sum1 : Sum  Inputs=++|
  c : Constant  Value=4200
  rho : Constant  Value=1000
  pT_out : Outport
  T_out : Outport  Port=2
  wires:
  Push/1(OutPot) -> Bus Selector/1
  Sum/1 -> Bus Creator1/2  "p"
  Gain/1 -> Sum/2
  Pull/2(OutFlow) -> Push/2(InFlow), Gain1/1, Product/2  "q"
  Gain1/1 -> Gain/1
  Pull/1(OutPot) -> pT_out/1
  pT_in/1 -> Push/1(InPot)
  Bus Selector/2 -> Sum/1  "<p>"
  Bus Creator1/1 -> Pull/1(InPot)
  Pull1/1 -> T_out/1  "T"
  Bus Selector/1 -> Sum1/2, Pull1/1  "<T>"
  Sum1/1 -> Bus Creator1/1  "T"
  Product/1 -> Sum1/1
  Pull1/2 -> Product/1
  c/1 -> Product/3
  rho/1 -> Product/4

== system Simple_lib/Hydraulic/Heat Sink/Linear Heat Pipe2 ==
  note: \Delta T = Q / (qc\rho))
  note: \Delta p = - k q
  pT_in : Inport
  Bus Creator1 : BusCreator  Inputs=2
  Bus Selector : BusSelector  OutputSignals=T,p
  Gain : Gain  Gain=-1
  Gain1 : Gain  Gain=1e3
  Product : Product  Inputs=*///
  Pull : Subsystem  Tag=Electrical  AncestorBlock=PlantUtilityBlockset_lib/Utility/Pull  InitFcn=initDuplex
      mask Display:
      | color('white')
      | plot([0 3], [2 2])
      | plot([0 3], [-2 -2])
      | color('black')
      | 
      | plot([0 1 1], [0 0 0.4])
      | plot([1 1 3], [0.6 1 1])
      | plot([1 3 2 1 0 2], [0.6 0.6 0.4 0.6 0.4 0.4])
      | patch([0 2 1],[0.4 0.4 0.6],[0,0,0])
      | plot([3 2 2], [1 1 0.6])
      | plot([2 2 3], [0.4 -1 -1])
  Pull1 : PlantUtilityBlockset_lib/Hydraulic/Linear Heat Pipe/Pull  Tag=Electrical  SystemSampleTime=-1
  Push : Subsystem  AncestorBlock=PlantUtilityBlockset_lib/Utility/Push  InitFcn=initSimplex
      mask Display:
      | color('white')
      | plot([0 3], [2 2])
      | plot([0 3], [-2 -2])
      | color('black')
      | 
      | plot([0 2 2 3], [1 1 0 0])
      | plot([1 3 2 1 0 2], [0.6 0.6 0.4 0.6 0.4 0.4])
      | patch([1 3 2],[0.6 0.6 0.4],[0,0,0])
      | plot([0 1 1], [1 1 0.6])
      | plot([1 1 0], [0.4 -1 -1])
  Sum : Sum  Inputs=|++
  Sum1 : Sum  Inputs=++|
  c : Constant  Value=4200
  rho : Constant  Value=1000
  pT_out : Outport
  T_out : Outport  Port=2
  wires:
  Push/1(OutPot) -> Bus Selector/1
  Sum/1 -> Bus Creator1/2  "p"
  Gain/1 -> Sum/2
  Pull/2(OutFlow) -> Push/2(InFlow), Gain1/1, Product/2  "q"
  Gain1/1 -> Gain/1
  Pull/1(OutPot) -> pT_out/1
  pT_in/1 -> Push/1(InPot)
  Bus Selector/2 -> Sum/1  "<p>"
  Bus Creator1/1 -> Pull/1(InPot)
  Pull1/1 -> T_out/1  "T"
  Bus Selector/1 -> Sum1/2, Pull1/1  "<T>"
  Sum1/1 -> Bus Creator1/1  "T"
  Product/1 -> Sum1/1
  Pull1/2 -> Product/1
  c/1 -> Product/3
  rho/1 -> Product/4

== system Simple_lib/Hydraulic/Heat Sink/Linear Heat Pipe3 ==
  note: \Delta T = Q / (qc\rho))
  note: \Delta p = - k q
  pT_in : Inport
  Bus Creator1 : BusCreator  Inputs=2
  Bus Selector : BusSelector  OutputSignals=T,p
  Gain : Gain  Gain=-1
  Gain1 : Gain  Gain=1e3
  Product : Product  Inputs=*///
  Pull : Subsystem  Tag=Electrical  AncestorBlock=PlantUtilityBlockset_lib/Utility/Pull  InitFcn=initDuplex
      mask Display:
      | color('white')
      | plot([0 3], [2 2])
      | plot([0 3], [-2 -2])
      | color('black')
      | 
      | plot([0 1 1], [0 0 0.4])
      | plot([1 1 3], [0.6 1 1])
      | plot([1 3 2 1 0 2], [0.6 0.6 0.4 0.6 0.4 0.4])
      | patch([0 2 1],[0.4 0.4 0.6],[0,0,0])
      | plot([3 2 2], [1 1 0.6])
      | plot([2 2 3], [0.4 -1 -1])
  Pull1 : PlantUtilityBlockset_lib/Hydraulic/Linear Heat Pipe/Pull  Tag=Electrical  SystemSampleTime=-1
  Push : Subsystem  AncestorBlock=PlantUtilityBlockset_lib/Utility/Push  InitFcn=initSimplex
      mask Display:
      | color('white')
      | plot([0 3], [2 2])
      | plot([0 3], [-2 -2])
      | color('black')
      | 
      | plot([0 2 2 3], [1 1 0 0])
      | plot([1 3 2 1 0 2], [0.6 0.6 0.4 0.6 0.4 0.4])
      | patch([1 3 2],[0.6 0.6 0.4],[0,0,0])
      | plot([0 1 1], [1 1 0.6])
      | plot([1 1 0], [0.4 -1 -1])
  Sum : Sum  Inputs=|++
  Sum1 : Sum  Inputs=++|
  c : Constant  Value=4200
  rho : Constant  Value=1000
  pT_out : Outport
  T_out : Outport  Port=2
  wires:
  Push/1(OutPot) -> Bus Selector/1
  Sum/1 -> Bus Creator1/2  "p"
  Gain/1 -> Sum/2
  Pull/2(OutFlow) -> Push/2(InFlow), Gain1/1, Product/2  "q"
  Gain1/1 -> Gain/1
  Pull/1(OutPot) -> pT_out/1
  pT_in/1 -> Push/1(InPot)
  Bus Selector/2 -> Sum/1  "<p>"
  Bus Creator1/1 -> Pull/1(InPot)
  Pull1/1 -> T_out/1  "T"
  Bus Selector/1 -> Sum1/2, Pull1/1  "<T>"
  Sum1/1 -> Bus Creator1/1  "T"
  Product/1 -> Sum1/1
  Pull1/2 -> Product/1
  c/1 -> Product/3
  rho/1 -> Product/4

== system Simple_lib/Hydraulic/Heat Sink/R1 ==
  In1 : Inport
  In2 : Inport  Port=2
  1/R1 : Gain  Gain=-1
  1/R2 : Gain  Gain=-1
  Discrete-Time Integrator1 : DiscreteIntegrator  gainval=1/10/Ts  SampleTime=Ts  ICPrevOutput=DiscIntNeverNeededParam  ICPrevScaledInput=DiscIntNeverNeededParam
  Simplex : Subsystem  Tag=Electrical  AncestorBlock=PlantUtilityBlockset_lib/Utility/Simplex  InitFcn=initSimplex
      mask Display:
      | color('white')
      | plot([0 3], [2 2])
      | plot([0 3], [-2 -2])
      | color('black')
      | 
      | plot([0 2 2 3], [1 1 0 0])
      | plot([1 3 2 1 0 2], [0.6 0.6 0.4 0.6 0.4 0.4])
      | patch([1 3 2],[0.6 0.6 0.4],[0,0,0])
      | plot([0 1 1], [1 1 0.6])
      | plot([1 1 0], [0.4 -1 -1])
  Simplex1 : Subsystem  Tag=Electrical  AncestorBlock=PlantUtilityBlockset_lib/Utility/Simplex  InitFcn=initSimplex
      mask Display:
      | color('white')
      | plot([0 3], [2 2])
      | plot([0 3], [-2 -2])
      | color('black')
      | 
      | plot([0 2 2 3], [1 1 0 0])
      | plot([1 3 2 1 0 2], [0.6 0.6 0.4 0.6 0.4 0.4])
      | patch([1 3 2],[0.6 0.6 0.4],[0,0,0])
      | plot([0 1 1], [1 1 0.6])
      | plot([1 1 0], [0.4 -1 -1])
  Sum : Sum  Inputs=+|+
  Sum1 : Sum  Inputs=|+-
  conductance : Gain  Gain=1/R
  wires:
  conductance/1 -> Sum1/1
  In1/1 -> Simplex/1(InPot)
  Simplex/1(OutPot) -> 1/R2/1
  1/R2/1 -> Sum/1
  Sum/1 -> conductance/1
  In2/1 -> Simplex1/1(InPot)
  Simplex1/1(OutPot) -> Sum/2
  1/R1/1 -> Simplex1/2(InFlow)
  Sum1/1 -> Discrete-Time Integrator1/1
  Discrete-Time Integrator1/1 -> Simplex/2(InFlow), 1/R1/1, Sum1/2

== system Simple_lib/Hydraulic/Isothermal Accumulator/Duplex ==
  InPot : Inport  Tag=NOFLUX
  FlowDisplay : Display
  FlowGain : Gain
  Flow_DuplexDivelineDoubleClutch1 : Scope
      settings: Tag=Flow
  PotDisplay : Display
  Pot_DuplexDivelineDoubleClutch1 : Scope
      settings: Tag=Pot
  Rate Transition : RateTransition  OutPortSampleTimeOpt=Multiple of input port sample time  OutPortSampleTimeMultiple=nT
  OutPot : Outport
  OutFlow : Outport  Tag=NOFLUX  Port=2
  wires:
  Rate Transition/1 -> OutPot/1
  InPot/1 -> Rate Transition/1, PotDisplay/1, Pot_DuplexDivelineDoubleClutch1/1
  FlowGain/1 -> OutFlow/1, Flow_DuplexDivelineDoubleClutch1/1, FlowDisplay/1

== system Simple_lib/Hydraulic/Isothermal Pump/PushBack ==
  InPot : Inport
  InFlow : Inport  Tag=NOFLUX  Port=2
  FlowDisplay : Display
  Flow_PushBackVacuumPumpFessSchematicSimulink : Scope
      settings: Tag=Flow
  PotDisplay : Display
  Pot_PushBackVacuumPumpFessSchematicSimulink : Scope
      settings: Tag=Pot
  Rate Transition : RateTransition  OutPortSampleTimeMultiple=Ts  OutPortSampleTime=Ts
  OutPot : Outport  Tag=NOFLUX
  tag scope: PushBackVacuumPumpFessSchematicSimulink=global
  wires:
  InPot/1 -> Rate Transition/1
  InFlow/1 -> Flow_PushBackVacuumPumpFessSchematicSimulink/1, FlowDisplay/1, [PushBackVacuumPumpFessSchematicSimulink]
  Rate Transition/1 -> OutPot/1, Pot_PushBackVacuumPumpFessSchematicSimulink/1, PotDisplay/1

== system Simple_lib/Hydraulic/Isothermal Pump/PushBack1 ==
  InPot : Inport
  InFlow : Inport  Tag=NOFLUX  Port=2
  FlowDisplay : Display
  Flow_PushBack1VacuumPumpFessSchematicSimulink : Scope
      settings: Tag=Flow
  PotDisplay : Display
  Pot_PushBack1VacuumPumpFessSchematicSimulink : Scope
      settings: Tag=Pot
  Rate Transition : RateTransition  OutPortSampleTimeMultiple=Ts  OutPortSampleTime=Ts
  OutPot : Outport  Tag=NOFLUX
  tag scope: PushBack1VacuumPumpFessSchematicSimulink=global
  wires:
  InPot/1 -> Rate Transition/1
  InFlow/1 -> Flow_PushBack1VacuumPumpFessSchematicSimulink/1, FlowDisplay/1, [PushBack1VacuumPumpFessSchematicSimulink]
  Rate Transition/1 -> OutPot/1, Pot_PushBack1VacuumPumpFessSchematicSimulink/1, PotDisplay/1

== system Simple_lib/Hydraulic/Isothermal Pump/PushBack2 ==
  InPot : Inport
  InFlow : Inport  Tag=NOFLUX  Port=2
  FlowDisplay : Display
  Flow_PushBack2VacuumPumpFessSchematicSimulink : Scope
      settings: Tag=Flow
  PotDisplay : Display
  Pot_PushBack2VacuumPumpFessSchematicSimulink : Scope
      settings: Tag=Pot
  Rate Transition : RateTransition  OutPortSampleTimeMultiple=Ts  OutPortSampleTime=Ts
  OutPot : Outport  Tag=NOFLUX
  tag scope: PushBack2VacuumPumpFessSchematicSimulink=global
  wires:
  InPot/1 -> Rate Transition/1
  InFlow/1 -> Flow_PushBack2VacuumPumpFessSchematicSimulink/1, FlowDisplay/1, [PushBack2VacuumPumpFessSchematicSimulink]
  Rate Transition/1 -> OutPot/1, Pot_PushBack2VacuumPumpFessSchematicSimulink/1, PotDisplay/1

== system Simple_lib/Hydraulic/Linear Heat Pipe/Pull ==
  InPot : Inport  Tag=NOFLUX
  FlowDisplay : Display
  FlowGain : Gain
  FlowSum : Sum  Inputs=2  SaturateOnIntegerOverflow=on  InputSameDT=on  OutDataTypeStr=Inherit: Same as first input
  Flow_PullO1BoxIIValveHydroNonStandard : Scope
      settings: Tag=Flow
  PotDisplay : Display
  Pot_PullO1BoxIIValveHydroNonStandard : Scope
      settings: Tag=Pot
  Rate Transition : RateTransition  OutPortSampleTimeMultiple=nT  OutPortSampleTime=Ts
  OutPot : Outport
  OutFlow : Outport  Tag=NOFLUX  Port=2
  wires:
  Rate Transition/1 -> OutPot/1
  InPot/1 -> Rate Transition/1, PotDisplay/1, Pot_PullO1BoxIIValveHydroNonStandard/1
  FlowGain/1 -> OutFlow/1, Flow_PullO1BoxIIValveHydroNonStandard/1, FlowDisplay/1
  FlowSum/1 -> FlowGain/1
  [PushO3BoxXValveHydroNonStandard] -> FlowSum/1
  [PushInertiaChamber1CylinderHydroNonStandard] -> FlowSum/2

== system Simple_lib/Hydraulic/Linear Heat Pipe/Push ==
  InPot : Inport
  InFlow : Inport  Tag=NOFLUX  Port=2
  FlowDisplay : Display
  Flow_PushO1BoxIIValveHydroNonStandard : Scope
      settings: Tag=Flow
  PotDisplay : Display
  Pot_PushO1BoxIIValveHydroNonStandard : Scope
      settings: Tag=Pot
  Rate Transition : RateTransition  OutPortSampleTimeMultiple=Ts  OutPortSampleTime=Ts
  OutPot : Outport  Tag=NOFLUX
  tag scope: PushO1BoxIIValveHydroNonStandard=global
  wires:
  Rate Transition/1 -> PotDisplay/1, Pot_PushO1BoxIIValveHydroNonStandard/1, OutPot/1
  InFlow/1 -> [PushO1BoxIIValveHydroNonStandard], FlowDisplay/1, Flow_PushO1BoxIIValveHydroNonStandard/1
  InPot/1 -> Rate Transition/1

== system Simple_lib/Hydraulic/Linear Pipe/Pull ==
  InPot : Inport  Tag=NOFLUX
  FlowDisplay : Display
  FlowGain : Gain
  FlowSum : Sum  Inputs=2  SaturateOnIntegerOverflow=on  InputSameDT=on  OutDataTypeStr=Inherit: Same as first input
  Flow_PullO1BoxIIValveHydroNonStandard : Scope
      settings: Tag=Flow
  PotDisplay : Display
  Pot_PullO1BoxIIValveHydroNonStandard : Scope
      settings: Tag=Pot
  Rate Transition : RateTransition  OutPortSampleTimeMultiple=nT  OutPortSampleTime=Ts
  OutPot : Outport
  OutFlow : Outport  Tag=NOFLUX  Port=2
  wires:
  Rate Transition/1 -> OutPot/1
  InPot/1 -> Rate Transition/1, PotDisplay/1, Pot_PullO1BoxIIValveHydroNonStandard/1
  FlowGain/1 -> OutFlow/1, Flow_PullO1BoxIIValveHydroNonStandard/1, FlowDisplay/1
  FlowSum/1 -> FlowGain/1
  [PushO3BoxXValveHydroNonStandard] -> FlowSum/1
  [PushInertiaChamber1CylinderHydroNonStandard] -> FlowSum/2

== system Simple_lib/Hydraulic/Linear Pipe/Push ==
  InPot : Inport
  InFlow : Inport  Tag=NOFLUX  Port=2
  FlowDisplay : Display
  Flow_PushO1BoxIIValveHydroNonStandard : Scope
      settings: Tag=Flow
  PotDisplay : Display
  Pot_PushO1BoxIIValveHydroNonStandard : Scope
      settings: Tag=Pot
  Rate Transition : RateTransition  OutPortSampleTimeMultiple=Ts  OutPortSampleTime=Ts
  OutPot : Outport  Tag=NOFLUX
  tag scope: PushO1BoxIIValveHydroNonStandard=global
  wires:
  Rate Transition/1 -> PotDisplay/1, Pot_PushO1BoxIIValveHydroNonStandard/1, OutPot/1
  InFlow/1 -> [PushO1BoxIIValveHydroNonStandard], FlowDisplay/1, Flow_PushO1BoxIIValveHydroNonStandard/1
  InPot/1 -> Rate Transition/1

== system Simple_lib/Hydraulic/Motor/Inertia ==
  1/I : Gain  Gain=1/2
  Discrete-Time Integrator1 : DiscreteIntegrator  gainval=1  SampleTime=Ts  ICPrevOutput=DiscIntNeverNeededParam  ICPrevScaledInput=DiscIntNeverNeededParam
  Duplex : Subsystem  Tag=Driveline  AncestorBlock=PlantUtilityBlockset_lib/Utility/Duplex  InitFcn=initDuplex
      mask Display:
      | color('white')
      | plot([0 3], [2 2])
      | plot([0 3], [-2 -2])
      | color('black')
      | 
      | plot([0 1 1], [0 0 0.4])
      | plot([1 1 3], [0.6 1 1])
      | plot([1 3 2 1 0 2], [0.6 0.6 0.4 0.6 0.4 0.4])
      | patch([0 2 1],[0.4 0.4 0.6],[0,0,0])
      | plot([3 2 2], [1 1 0.6])
      | plot([2 2 3], [0.4 -1 -1])
  Out1 : Outport
  wires:
  Duplex/2(OutFlow) -> 1/I/1
  Duplex/1(OutPot) -> Out1/1
  1/I/1 -> Discrete-Time Integrator1/1
  Discrete-Time Integrator1/1 -> Duplex/1(InPot)

== system Simple_lib/Hydraulic/Motor/PushBack ==
  InPot : Inport
  InFlow : Inport  Tag=NOFLUX  Port=2
  FlowDisplay : Display
  Flow_PushBackMotor2FessSchematicSimulink : Scope
      settings: Tag=Flow
  PotDisplay : Display
  Pot_PushBackMotor2FessSchematicSimulink : Scope
      settings: Tag=Pot
  Rate Transition : RateTransition  OutPortSampleTimeMultiple=Ts  OutPortSampleTime=Ts
  OutPot : Outport  Tag=NOFLUX
  tag scope: PushBackMotor2FessSchematicSimulink=global
  wires:
  InPot/1 -> Rate Transition/1
  InFlow/1 -> Flow_PushBackMotor2FessSchematicSimulink/1, FlowDisplay/1, [PushBackMotor2FessSchematicSimulink]
  Rate Transition/1 -> OutPot/1, Pot_PushBackMotor2FessSchematicSimulink/1, PotDisplay/1

== system Simple_lib/Hydraulic/Pressure Meter/PushBack ==
  InPot : Inport
  InFlow : Inport  Tag=NOFLUX  Port=2
  FlowDisplay : Display
  Flow_PushBack1OilPumpFessSchematicSimulink : Scope
      settings: Tag=Flow
  PotDisplay : Display
  Pot_PushBack1OilPumpFessSchematicSimulink : Scope
      settings: Tag=Pot
  Rate Transition : RateTransition  OutPortSampleTimeMultiple=Ts  OutPortSampleTime=Ts
  OutPot : Outport  Tag=NOFLUX
  tag scope: PushBack1OilPumpFessSchematicSimulink=global
  wires:
  Rate Transition/1 -> PotDisplay/1, Pot_PushBack1OilPumpFessSchematicSimulink/1, OutPot/1
  InFlow/1 -> [PushBack1OilPumpFessSchematicSimulink], FlowDisplay/1, Flow_PushBack1OilPumpFessSchematicSimulink/1
  InPot/1 -> Rate Transition/1

== system Simple_lib/Hydraulic/Quadratic Heat Pipe/Pull ==
  InPot : Inport  Tag=NOFLUX
  FlowDisplay : Display
  FlowGain : Gain
  FlowSum : Sum  Inputs=2  SaturateOnIntegerOverflow=on  InputSameDT=on  OutDataTypeStr=Inherit: Same as first input
  Flow_PullO1BoxIIValveHydroNonStandard : Scope
      settings: Tag=Flow
  PotDisplay : Display
  Pot_PullO1BoxIIValveHydroNonStandard : Scope
      settings: Tag=Pot
  Rate Transition : RateTransition  OutPortSampleTimeMultiple=nT  OutPortSampleTime=Ts
  OutPot : Outport
  OutFlow : Outport  Tag=NOFLUX  Port=2
  wires:
  Rate Transition/1 -> OutPot/1
  InPot/1 -> Rate Transition/1, PotDisplay/1, Pot_PullO1BoxIIValveHydroNonStandard/1
  FlowGain/1 -> OutFlow/1, Flow_PullO1BoxIIValveHydroNonStandard/1, FlowDisplay/1
  FlowSum/1 -> FlowGain/1
  [PushO3BoxXValveHydroNonStandard] -> FlowSum/1
  [PushInertiaChamber1CylinderHydroNonStandard] -> FlowSum/2
